simulink model "ESC"  (R2013a)
settings: Solver=ode45  SolverMode=SingleTasking  StartTime=0.0  StopTime=MOD.tFinal  FixedStep=1e-6  MinStep=9e-9  RelTol=0.001
PreLoadFcn:
  | setPath
  | eval(sprintf('PreLoadFcn_%s', gcs))
  | eval(sprintf('InitFcn_%s', gcs))
InitFcn:
  | eval(sprintf('InitFcn_%s', gcs))
StopFcn:
  | eval(sprintf('StopFcn_%s', gcs))
undefined symbols (not defined in the file or in its folder): E, ic, ln, MOD
libraries: simulink x1
settings Model: Creator=210023782  LastModifiedBy=210023782
settings SolverCC: InitialStep=1e-7  MaxConsecutiveMinStep=1000000  ZeroCrossControl=DisableAll
settings DebuggingCC: AlgebraicLoopMsg=error  CheckSSInitialOutputMsg=off  SolverPrmCheckMsg=none  InheritedTsInSrcMsg=none  MultiTaskRateTransMsg=warning
settings ModelReferenceCC: UpdateModelReferenceTargets=IfOutOfDate
settings SFSimCC: SFSimEcho=off

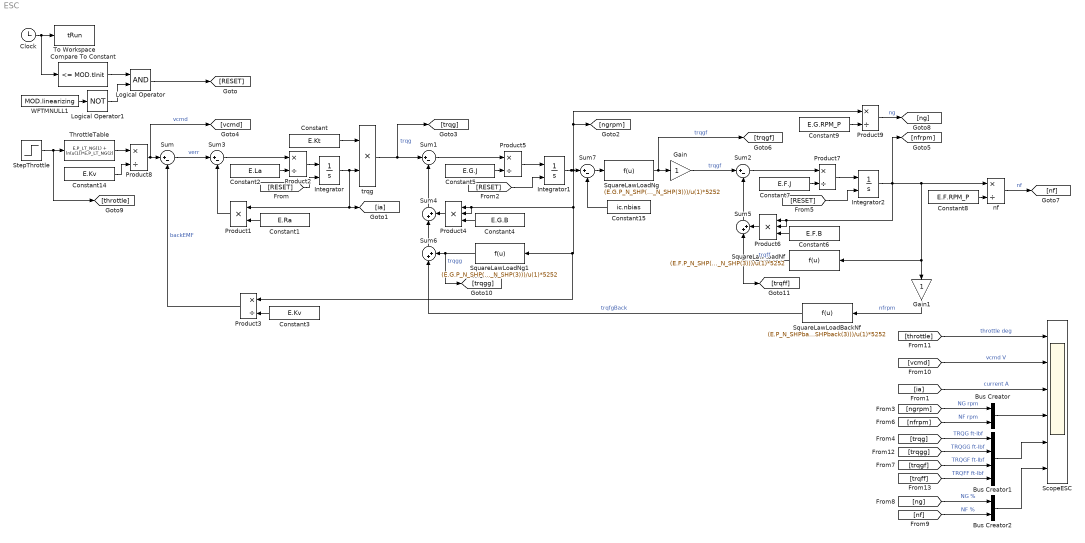
== system ESC ==
  Bus Creator : BusCreator  Inputs=2
  Bus Creator1 : BusCreator
  Bus Creator2 : BusCreator  Inputs=2
  Clock : Clock
  Compare To Constant : simulink/Logic and Bit Operations/Compare To Constant  relop=<=  const=MOD.tInit  OutDataTypeStr=boolean
  Constant : Constant  Value=E.Kt
  Constant1 : Constant  Value=E.Ra
  Constant14 : Constant  Value=E.Kv
  Constant15 : Constant  Value=ic.nbias
  Constant2 : Constant  Value=E.La
  Constant3 : Constant  Value=E.Kv
  Constant4 : Constant  Value=E.G.B
  Constant5 : Constant  Value=E.G.J
  Constant6 : Constant  Value=E.F.B
  Constant7 : Constant  Value=E.F.J
  Constant8 : Constant  Value=E.F.RPM_P
  Constant9 : Constant  Value=E.G.RPM_P
  Gain : Gain
  Gain1 : Gain
  Integrator : Integrator  ExternalReset=level  InitialCondition=ic.ia
  Integrator1 : Integrator  ExternalReset=level  InitialCondition=ic.E.G.nrpm
  Integrator2 : Integrator  ExternalReset=level  InitialCondition=ic.E.F.nrpm
  Logical Operator : Logic  AllPortsSameDT=off  OutDataTypeStr=boolean
  Logical Operator1 : Logic  Operator=NOT  AllPortsSameDT=off  OutDataTypeStr=boolean
  Product1 : Product
  Product{2..3,5,7..9} (6 alike) : Product  Inputs=*/
  Product4 : Product  Inputs=3
  Product6 : Product  Inputs=3
  ScopeESC : Scope  NumInputPorts=6
      settings: ShowLegends=on  YMin=-5~-5~-5~-5~-5~-5  YMax=5~5~5~5~5~5
  SquareLawLoadBackNf : Fcn  Expr=(E.P_N_SHPback(1) + u(1)*(E.P_N_SHPback(2)+ u(1)*E.P_N_SHPback(3)))/u(1)*5252
  SquareLawLoadNf : Fcn  Expr=(E.F.P_N_SHP(1) + u(1)*(E.F.P_N_SHP(2)+ u(1)*E.F.P_N_SHP(3)))/u(1)*5252
  SquareLawLoadNg : Fcn  Expr=(E.G.P_N_SHP(1) + u(1)*(E.G.P_N_SHP(2)+ u(1)*E.G.P_N_SHP(3)))/u(1)*5252
  SquareLawLoadNg1 : Fcn  Expr=(E.G.P_N_SHP(1) + u(1)*(E.G.P_N_SHP(2)+ u(1)*E.G.P_N_SHP(3)))/u(1)*5252
  StepThrottle : Step  Time=MOD.tStep  Before=ic.throttle  After=ic.throttle+10  SampleTime=E.Tminor
  Sum{,1..3,7} (5 alike) : Sum  Inputs=|+-
  Sum4 : Sum  Inputs=|++
  Sum5 : Sum  Inputs=|++
  Sum6 : Sum  Inputs=|++
  ThrottleTable : Fcn  Expr=E.P_LT_NG(1) + ln(u(1))*E.P_LT_NG(2)
  To Workspace : ToWorkspace  VariableName=tRun  SampleTime=-1  SaveFormat=Timeseries
  WFTMNULL1 : Constant  Value=MOD.linearizing  OutDataTypeStr=double
  nf : Product  Inputs=*/
  trqg : Product
  wires:
  Clock/1 -> Compare To Constant/1, To Workspace/1
  Constant/1 -> trqg/1
  Constant1/1 -> Product1/2
  Product1/1 -> Sum3/2
  Product2/1 -> Integrator/1
  Constant2/1 -> Product2/2
  [RESET] -> Integrator/2
  Integrator/1 -> [ia], Product1/1, trqg/2
  Sum/1 -> Sum3/1  "verr"
  Constant3/1 -> Product3/2
  trqg/1 -> [trqg], Sum1/1  "trqg"
  Sum4/1 -> Sum1/2
  Product4/1 -> Sum4/2
  Integrator1/1 -> Product9/1, [ngrpm], Product4/2, Product4/1, SquareLawLoadNg1/1, Product3/1, Sum7/1
  Sum1/1 -> Product5/1
  Constant5/1 -> Product5/2
  Product5/1 -> Integrator1/1
  [RESET] -> Integrator1/2
  Product3/1 -> Sum/2  "backEMF"
  Sum5/1 -> Sum2/2
  Product6/1 -> Sum5/2
  Sum2/1 -> Product7/1
  Constant7/1 -> Product7/2
  Product7/1 -> Integrator2/1
  [RESET] -> Integrator2/2
  Constant8/1 -> nf/2
  nf/1 -> [nf]  "nf"
  Constant9/1 -> Product9/2
  Product9/1 -> [ng]  "ng"
  Constant4/1 -> Product4/3
  [vcmd] -> ScopeESC/2  "vcmd V"
  [ia] -> ScopeESC/3  "current A"
  Bus Creator/1 -> ScopeESC/4
  [ngrpm] -> Bus Creator/1  "NG rpm"
  [nfrpm] -> Bus Creator/2  "NF rpm"
  [trqg] -> Bus Creator1/1  "TRQG ft-lbf"
  [trqgf] -> Bus Creator1/3  "TRQGF ft-lbf"
  [nf] -> Bus Creator2/2  "NF %"
  [ng] -> Bus Creator2/1  "NG %"
  Bus Creator2/1 -> ScopeESC/6
  SquareLawLoadNg/1 -> Gain/1, [trqgf]  "trqgf"
  Sum6/1 -> Sum4/1
  SquareLawLoadNf/1 -> [trqff], Sum5/1  "trqff"
  Constant6/1 -> Product6/3
  Integrator2/1 -> [nfrpm], Product6/2, Product6/1, nf/1, SquareLawLoadNf/1, Gain1/1
  Logical Operator/1 -> [RESET]
  Logical Operator1/1 -> Logical Operator/2
  WFTMNULL1/1 -> Logical Operator1/1
  Gain/1 -> Sum2/1  "trqgf"
  Gain1/1 -> SquareLawLoadBackNf/1  "nfrpm"
  ThrottleTable/1 -> Product8/1
  Constant14/1 -> Product8/2
  Product8/1 -> [vcmd], Sum/1  "vcmd"
  StepThrottle/1 -> [throttle], ThrottleTable/1
  Bus Creator1/1 -> ScopeESC/5
  [throttle] -> ScopeESC/1  "throttle deg"
  SquareLawLoadBackNf/1 -> Sum6/1  "trqfgBack"
  SquareLawLoadNg1/1 -> [trqgg], Sum6/2  "trqgg"
  Sum7/1 -> SquareLawLoadNg/1
  Constant15/1 -> Sum7/2
  [trqgg] -> Bus Creator1/2  "TRQGG ft-lbf"
  [trqff] -> Bus Creator1/4  "TRQFF ft-lbf"
  Compare To Constant/1 -> Logical Operator/1
  Sum3/1 -> Product2/1
